simulink model "circuit1"  (R2020b)
settings: Solver=VariableStepAuto  StartTime=0.0  StopTime=10.0  RelTol=1e-3
settings Model: Creator=sushma  LastModifiedBy=sushma

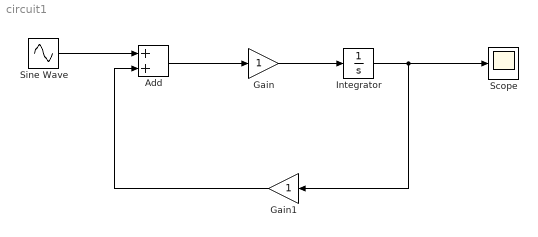
== system circuit1 ==
  Add : Sum
  Gain : Gain
  Gain1 : Gain
  Integrator : Integrator
  Scope : Scope
  Sine Wave : Sin  SampleTime=0
  wires:
  Sine Wave/1 -> Add/1
  Add/1 -> Gain/1
  Gain/1 -> Integrator/1
  Integrator/1 -> Gain1/1, Scope/1
  Gain1/1 -> Add/2
